simulink model "example_House_RoomRadiator"  (R2013b)
settings: Solver=ode23t  StartTime=0.0  StopTime=24*3600  RelTol=1e-3
libraries: carnot x6
settings Model: Creator=drhf  LastModifiedBy=drhf
settings OptimizationCC: ExpressionDepthLimit=2147483647
settings DebuggingCC: StateNameClashWarn=warning
settings GRTTargetCC: CombineOutputUpdateFcns=off  GRTInterface=on

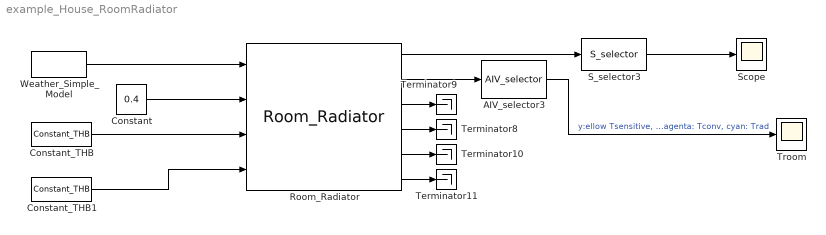
== system example_House_RoomRadiator ==
  AIV_selector3 : carnot/Outputs/AIV_selector  e1=on  e2=on  e3=on  e4=off  e5=off  e6=off  e7=off  e8=off  e9=off
  Constant : Constant  Value=0.4
  Constant_THB : carnot/Source/Simple/Constant_THB  t=30  mdot=600/3600  p=1e5  mID=No Pressure Drop  fluid=Water  mix=0  dia=0.02  hgt=0
  Constant_THB1 : carnot/Source/Simple/Constant_THB  t=40  mdot=600/3600  p=1e5  mID=No Pressure Drop  fluid=Water  mix=0  dia=0.02  hgt=0
  Room_Radiator : carnot/Load/Houses/Room_Radiator  t0=20  temp_neighbour=20
  S_selector3 : carnot/Outputs/S_selector  e1=off  e2=off  e3=off  e4=off  e5=off  e6=off  e7=on  e8=on  e9=off  e10=off  e11=off  e12=off  e13=off
  Scope : Scope
      settings: YMin=0  YMax=12
  Terminator{8..11} (4 alike) : Terminator
  Troom : Scope
  Weather_Simple_Model : carnot/Weather/Weather_Simple_Model  lat=60  Ibn=900  Idg=100  tamb=5  deltaTsky=-6  rh=50  precip="10e-3/24/3600           % 10 mm in 24 h"  cloud=0.125  p=1013e2  vw=1  wdir=270
  wires:
  Weather_Simple_Model/1 -> Room_Radiator/1
  Constant/1 -> Room_Radiator/2
  Constant_THB/1 -> Room_Radiator/3
  Constant_THB1/1 -> Room_Radiator/4
  Room_Radiator/4 -> Terminator8/1
  Room_Radiator/3 -> Terminator9/1
  Room_Radiator/5 -> Terminator10/1
  Room_Radiator/6 -> Terminator11/1
  Room_Radiator/2 -> AIV_selector3/1
  Room_Radiator/1 -> S_selector3/1
  S_selector3/1 -> Scope/1
  AIV_selector3/1 -> Troom/1  "y:ellow Tsensitive, magenta: Tconv, cyan: Trad"
